simulink model "mod_simple"  (R2014a)
settings: Solver=ode45  StartTime=0.0  StopTime=10.0  RelTol=1e-3
undefined symbols (not defined in the file): b, K, mu_max, Qn, Qp, Si, V, Y
settings Model: Creator=Tanay  LastModifiedBy=Tanay

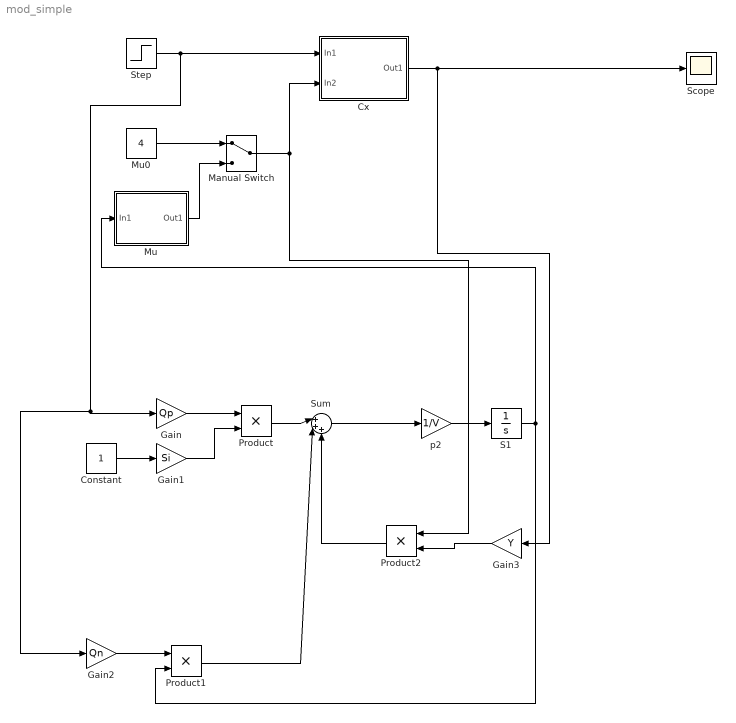
== system mod_simple ==
  Constant : Constant
  Cx : Subsystem
  Gain : Gain  Gain=Qp
  Gain1 : Gain  Gain=Si
  Gain2 : Gain  Gain=Qn
  Gain3 : Gain  Gain=Y
  Manual Switch : ManualSwitch
  Mu : Subsystem
  Mu0 : Constant  Value=4
  Product : Product
  Product1 : Product
  Product2 : Product
  S1 : Integrator
  Scope : Scope
  Step : Step  SampleTime=0
  Sum : Sum  Inputs=|+++
  p2 : Gain  Gain=1/V
  wires:
  p2/1 -> S1/1
  Manual Switch/1 -> Cx/2(In2), Product2/1
  Mu0/1 -> Manual Switch/1
  Mu/1(Out1) -> Manual Switch/2
  Sum/1 -> p2/1
  Gain/1 -> Product/1
  Gain1/1 -> Product/2
  Product/1 -> Sum/1
  Constant/1 -> Gain1/1
  Gain2/1 -> Product1/1
  S1/1 -> Mu/1(In1), Product1/2
  Product1/1 -> Sum/2
  Step/1 -> Gain2/1, Gain/1, Cx/1(In1)
  Cx/1(Out1) -> Gain3/1, Scope/1
  Gain3/1 -> Product2/2
  Product2/1 -> Sum/3

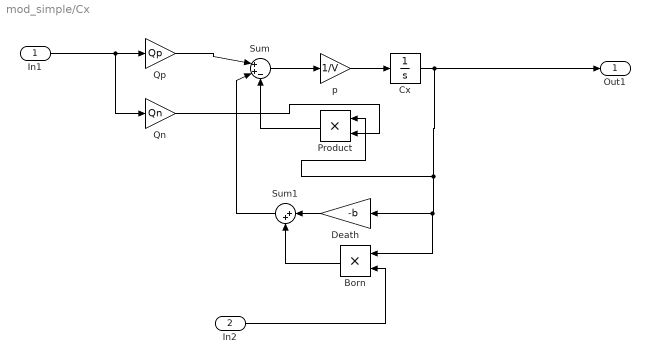
== system mod_simple/Cx ==
  In1 : Inport
  In2 : Inport  Port=2
  Born : Product
  Cx : Integrator
  Death : Gain  Gain=-b
  Product : Product
  Qn : Gain  Gain=Qn
  Qp : Gain  Gain=Qp
  Sum : Sum  Inputs=|++-
  Sum1 : Sum  Inputs=|++
  p : Gain  Gain=1/V
  Out1 : Outport
  wires:
  In2/1 -> Born/2
  p/1 -> Cx/1
  In1/1 -> Qn/1, Qp/1
  Sum/1 -> p/1
  Born/1 -> Sum1/2
  Qn/1 -> Product/2
  Sum1/1 -> Sum/2
  Qp/1 -> Sum/1
  Death/1 -> Sum1/1
  Cx/1 -> Out1/1, Born/1, Death/1, Product/1
  Product/1 -> Sum/3

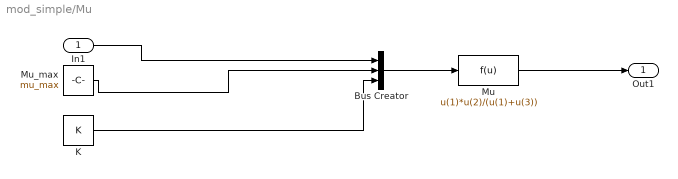
== system mod_simple/Mu ==
  In1 : Inport
  Bus Creator : BusCreator  Inputs=3
  K : Constant  Value=K
  Mu : Fcn  Expr=u(1)*u(2)/(u(1)+u(3))
  Mu_max : Constant  Value=mu_max
  Out1 : Outport
  wires:
  Mu_max/1 -> Bus Creator/2
  Mu/1 -> Out1/1
  In1/1 -> Bus Creator/1
  K/1 -> Bus Creator/3
  Bus Creator/1 -> Mu/1
